simulink model "SecRwLtStBkReclnTrgtPosSelc"  (R2018b)
settings: Solver=FixedStepDiscrete  StartTime=0.0  StopTime=10.0  FixedStep=0.01  RelTol=1e-3
undefined symbols (not defined in the file): KeSMSw4SAcsMd21SecRwLtStBkReclnUpwdDnwdPos_Val, KeSMSw4SAcsMd21SecRwLtStBkReclnUpwdDnwdPosMax_Val, KeSMSw4SAcsMd21SecRwLtStBkReclnUpwdDnwdPosMin_Val, KeSMSw4SAcsMd22SecRwLtStBkReclnUpwdDnwdPos1_Val, KeSMSw4SAcsMd22SecRwLtStBkReclnUpwdDnwdPos1Max_Val, KeSMSw4SAcsMd22SecRwLtStBkReclnUpwdDnwdPos1Min_Val, KeSMSw4SAcsMd22SecRwLtStBkReclnUpwdDnwdPos2_Val, KeSMSw4SAcsMd22SecRwLtStBkReclnUpwdDnwdPos2Max_Val, KeSMSw4SAcsMd22SecRwLtStBkReclnUpwdDnwdPos2Min_Val, KeSMSw4SAcsMd25SecRwLtStBkReclnUpwdDnwdPos_Val, KeSMSw4SAcsMd25SecRwLtStBkReclnUpwdDnwdPosMax_Val, KeSMSw4SAcsMd25SecRwLtStBkReclnUpwdDnwdPosMin_Val, KeSMSw4SAcsMd26SecRwLtStBkReclnUpwdDnwdPos_Val, KeSMSw4SAcsMd26SecRwLtStBkReclnUpwdDnwdPosMax_Val, KeSMSw4SAcsMd26SecRwLtStBkReclnUpwdDnwdPosMin_Val, KeSMSw4sLyingMDSecRwLtStBkReclnUpwdDnwdPos_Val, KeSMSw4sLyingMDSecRwLtStBkReclnUpwdDnwdPosMax_Val, KeSMSw4sLyingMDSecRwLtStBkReclnUpwdDnwdPosMin_Val, KeSMSw4sRecoveryMDSecRwLtStBkReclnUpwdDnwdPos_Val, KeSMSw4sRecoveryMDSecRwLtStBkReclnUpwdDnwdPosMax_Val, KeSMSw4sRecoveryMDSecRwLtStBkReclnUpwdDnwdPosMin_Val, KeSMSw4sVIPMDSecRwLtStBkReclnUpwdDnwdPos_Val, KeSMSw4sVIPMDSecRwLtStBkReclnUpwdDnwdPosMax_Val, KeSMSw4sVIPMDSecRwLtStBkReclnUpwdDnwdPosMin_Val, KeSMSw6sAcsEntrySecRwLtStBkReclnUpwdDnwd1Pos_Val, KeSMSw6sAcsEntrySecRwLtStBkReclnUpwdDnwdPos1Max_Val, KeSMSw6sAcsEntrySecRwLtStBkReclnUpwdDnwdPos1Min_Val, KeSMSw6sAcsEntrySecRwLtStBkReclnUpwdDnwdPos_Val, KeSMSw6sAcsEntrySecRwLtStBkReclnUpwdDnwdPosMax_Val, KeSMSw6sAcsEntrySecRwLtStBkReclnUpwdDnwdPosMin_Val, KeSMSw6sAcsExtSecRwLtStBkReclnUpwdDnwdPos_Val, KeSMSw6sAcsExtSecRwLtStBkReclnUpwdDnwdPosMax_Val, KeSMSw6sAcsExtSecRwLtStBkReclnUpwdDnwdPosMin_Val, KeSMSw6sRecoveryMdSecRwLtStBkReclnUpwdDnwdPos_Val, KeSMSw6sRecoveryMdSecRwLtStBkReclnUpwdDnwdPosMax_Val, KeSMSw6sRecoveryMdSecRwLtStBkReclnUpwdDnwdPosMin_Val, KeSMSw6sVIPSecRwLtStBkReclnUpwdDnwdPos_Val, KeSMSw6sVIPSecRwLtStBkReclnUpwdDnwdPosMax_Val, KeSMSw6sVIPSecRwLtStBkReclnUpwdDnwdPosMin_Val, KeSMSwAcsEntrySecRwLtStBkReclnUpwdDnwdPos1_Val, KeSMSwAcsEntrySecRwLtStBkReclnUpwdDnwdPos1Max_Val, KeSMSwAcsEntrySecRwLtStBkReclnUpwdDnwdPos1Min_Val, KeSMSwAcsEntrySecRwLtStBkReclnUpwdDnwdPos_Val, KeSMSwAcsEntrySecRwLtStBkReclnUpwdDnwdPosMax_Val, KeSMSwAcsEntrySecRwLtStBkReclnUpwdDnwdPosMin_Val, KeSMSwAcsExtSecRwLtStBkReclnUpwdDnwdPos_Val, KeSMSwAcsExtSecRwLtStBkReclnUpwdDnwdPosMax_Val, KeSMSwAcsExtSecRwLtStBkReclnUpwdDnwdPosMin_Val, KeSMSwAcsMd32SecRwLtStBkReclnUpwdDnwdPos1_Val, KeSMSwAcsMd32SecRwLtStBkReclnUpwdDnwdPos1Max_Val, KeSMSwAcsMd32SecRwLtStBkReclnUpwdDnwdPos1Min_Val, KeSMSwAcsMd32SecRwLtStBkReclnUpwdDnwdPos_Val, KeSMSwAcsMd32SecRwLtStBkReclnUpwdDnwdPosMax_Val, KeSMSwAcsMd32SecRwLtStBkReclnUpwdDnwdPosMin_Val, KeSMSwAcsMd8SecRwLtStBkReclnUpwdDnwdPos_Val, KeSMSwAcsMd8SecRwLtStBkReclnUpwdDnwdPosMax_Val, KeSMSwAcsMd8SecRwLtStBkReclnUpwdDnwdPosMin_Val, KeSMSwRecoveryMdSecRwLtStBkReclnUpwdDnwdPos_Val, KeSMSwRecoveryMdSecRwLtStBkReclnUpwdDnwdPosMax_Val, KeSMSwRecoveryMdSecRwLtStBkReclnUpwdDnwdPosMin_Val ... (+3)
libraries: TrgtPosSelcLib x13, StIsPosChkLib x1, simulink x1
(part 2 of 2)

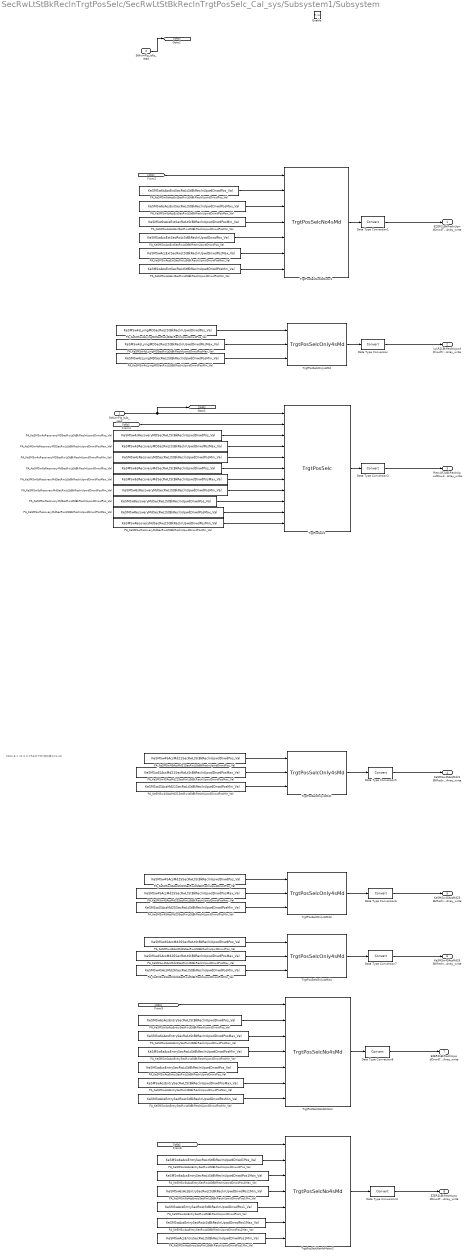
== system SecRwLtStBkReclnTrgtPosSelc/SecRwLtStBkReclnTrgtPosSelc_Cal_sys/Subsystem1/Subsystem ==
  note: 2023.8.1 V2.0.0 CR421790 增加模式21-26
  StNumFlg_Is4s_read : Inport
  StNumFlg_Is6s_read : Inport  Port=2
  Enable : EnablePort
  Data Type Conversion{,1..3,5..8} (8 alike) : DataTypeConversion
  PA_KeSMSw4SAcsMd21SecRwLtStBkReclnUpwdDnwdPosMax_Val : Constant  Value=KeSMSw4SAcsMd21SecRwLtStBkReclnUpwdDnwdPosMax_Val
  PA_KeSMSw4SAcsMd21SecRwLtStBkReclnUpwdDnwdPosMin_Val : Constant  Value=KeSMSw4SAcsMd21SecRwLtStBkReclnUpwdDnwdPosMin_Val
  PA_KeSMSw4SAcsMd21SecRwLtStBkReclnUpwdDnwdPos_Val : Constant  Value=KeSMSw4SAcsMd21SecRwLtStBkReclnUpwdDnwdPos_Val
  PA_KeSMSw4SAcsMd25SecRwLtStBkReclnUpwdDnwdPosMax_Val : Constant  Value=KeSMSw4SAcsMd25SecRwLtStBkReclnUpwdDnwdPosMax_Val
  PA_KeSMSw4SAcsMd25SecRwLtStBkReclnUpwdDnwdPosMin_Val : Constant  Value=KeSMSw4SAcsMd25SecRwLtStBkReclnUpwdDnwdPosMin_Val
  PA_KeSMSw4SAcsMd25SecRwLtStBkReclnUpwdDnwdPos_Val : Constant  Value=KeSMSw4SAcsMd25SecRwLtStBkReclnUpwdDnwdPos_Val
  PA_KeSMSw4SAcsMd26SecRwLtStBkReclnUpwdDnwdPosMax_Val : Constant  Value=KeSMSw4SAcsMd26SecRwLtStBkReclnUpwdDnwdPosMax_Val
  PA_KeSMSw4SAcsMd26SecRwLtStBkReclnUpwdDnwdPosMin_Val : Constant  Value=KeSMSw4SAcsMd26SecRwLtStBkReclnUpwdDnwdPosMin_Val
  PA_KeSMSw4SAcsMd26SecRwLtStBkReclnUpwdDnwdPos_Val : Constant  Value=KeSMSw4SAcsMd26SecRwLtStBkReclnUpwdDnwdPos_Val
  PA_KeSMSw4sLyingMDSecRwLtStBkReclnUpwdDnwdPosMax_Val : Constant  Value=KeSMSw4sLyingMDSecRwLtStBkReclnUpwdDnwdPosMax_Val
  PA_KeSMSw4sLyingMDSecRwLtStBkReclnUpwdDnwdPosMin_Val : Constant  Value=KeSMSw4sLyingMDSecRwLtStBkReclnUpwdDnwdPosMin_Val
  PA_KeSMSw4sLyingMDSecRwLtStBkReclnUpwdDnwdPos_Val : Constant  Value=KeSMSw4sLyingMDSecRwLtStBkReclnUpwdDnwdPos_Val
  PA_KeSMSw4sRecoveryMDSecRwLtStBkReclnUpwdDnwdPosMax_Val : Constant  Value=KeSMSw4sRecoveryMDSecRwLtStBkReclnUpwdDnwdPosMax_Val
  PA_KeSMSw4sRecoveryMDSecRwLtStBkReclnUpwdDnwdPosMin_Val : Constant  Value=KeSMSw4sRecoveryMDSecRwLtStBkReclnUpwdDnwdPosMin_Val
  PA_KeSMSw4sRecoveryMDSecRwLtStBkReclnUpwdDnwdPos_Val : Constant  Value=KeSMSw4sRecoveryMDSecRwLtStBkReclnUpwdDnwdPos_Val
  PA_KeSMSw6sAcsEntrySecRwLtStBkReclnUpwdDnwd1Pos_Val : Constant  Value=KeSMSw6sAcsEntrySecRwLtStBkReclnUpwdDnwd1Pos_Val
  PA_KeSMSw6sAcsEntrySecRwLtStBkReclnUpwdDnwdPos1Max_Val : Constant  Value=KeSMSw6sAcsEntrySecRwLtStBkReclnUpwdDnwdPos1Max_Val
  PA_KeSMSw6sAcsEntrySecRwLtStBkReclnUpwdDnwdPos1Min_Val : Constant  Value=KeSMSw6sAcsEntrySecRwLtStBkReclnUpwdDnwdPos1Min_Val
  PA_KeSMSw6sAcsEntrySecRwLtStBkReclnUpwdDnwdPosMax_Val : Constant  Value=KeSMSw6sAcsEntrySecRwLtStBkReclnUpwdDnwdPosMax_Val
  PA_KeSMSw6sAcsEntrySecRwLtStBkReclnUpwdDnwdPosMin_Val : Constant  Value=KeSMSw6sAcsEntrySecRwLtStBkReclnUpwdDnwdPosMin_Val
  PA_KeSMSw6sAcsEntrySecRwLtStBkReclnUpwdDnwdPos_Val : Constant  Value=KeSMSw6sAcsEntrySecRwLtStBkReclnUpwdDnwdPos_Val
  PA_KeSMSw6sAcsExtSecRwLtStBkReclnUpwdDnwdPosMax_Val : Constant  Value=KeSMSw6sAcsExtSecRwLtStBkReclnUpwdDnwdPosMax_Val
  PA_KeSMSw6sAcsExtSecRwLtStBkReclnUpwdDnwdPosMin_Val : Constant  Value=KeSMSw6sAcsExtSecRwLtStBkReclnUpwdDnwdPosMin_Val
  PA_KeSMSw6sAcsExtSecRwLtStBkReclnUpwdDnwdPos_Val : Constant  Value=KeSMSw6sAcsExtSecRwLtStBkReclnUpwdDnwdPos_Val
  PA_KeSMSw6sRecoveryMdSecRwLtStBkReclnUpwdDnwdPosMax_Val : Constant  Value=KeSMSw6sRecoveryMdSecRwLtStBkReclnUpwdDnwdPosMax_Val
  PA_KeSMSw6sRecoveryMdSecRwLtStBkReclnUpwdDnwdPosMin_Val : Constant  Value=KeSMSw6sRecoveryMdSecRwLtStBkReclnUpwdDnwdPosMin_Val
  PA_KeSMSw6sRecoveryMdSecRwLtStBkReclnUpwdDnwdPos_Val : Constant  Value=KeSMSw6sRecoveryMdSecRwLtStBkReclnUpwdDnwdPos_Val
  PA_KeSMSwAcsEntrySecRwLtStBkReclnUpwdDnwdPos1Max_Val : Constant  Value=KeSMSwAcsEntrySecRwLtStBkReclnUpwdDnwdPos1Max_Val
  PA_KeSMSwAcsEntrySecRwLtStBkReclnUpwdDnwdPos1Min_Val : Constant  Value=KeSMSwAcsEntrySecRwLtStBkReclnUpwdDnwdPos1Min_Val
  PA_KeSMSwAcsEntrySecRwLtStBkReclnUpwdDnwdPos1_Val : Constant  Value=KeSMSwAcsEntrySecRwLtStBkReclnUpwdDnwdPos1_Val
  PA_KeSMSwAcsEntrySecRwLtStBkReclnUpwdDnwdPosMax_Val : Constant  Value=KeSMSwAcsEntrySecRwLtStBkReclnUpwdDnwdPosMax_Val
  PA_KeSMSwAcsEntrySecRwLtStBkReclnUpwdDnwdPosMin_Val : Constant  Value=KeSMSwAcsEntrySecRwLtStBkReclnUpwdDnwdPosMin_Val
  PA_KeSMSwAcsEntrySecRwLtStBkReclnUpwdDnwdPos_Val : Constant  Value=KeSMSwAcsEntrySecRwLtStBkReclnUpwdDnwdPos_Val
  PA_KeSMSwAcsExtSecRwLtStBkReclnUpwdDnwdPosMax_Val : Constant  Value=KeSMSwAcsExtSecRwLtStBkReclnUpwdDnwdPosMax_Val
  PA_KeSMSwAcsExtSecRwLtStBkReclnUpwdDnwdPosMin_Val : Constant  Value=KeSMSwAcsExtSecRwLtStBkReclnUpwdDnwdPosMin_Val
  PA_KeSMSwAcsExtSecRwLtStBkReclnUpwdDnwdPos_Val : Constant  Value=KeSMSwAcsExtSecRwLtStBkReclnUpwdDnwdPos_Val
  PA_KeSMSwRecoveryMdSecRwLtStBkReclnUpwdDnwdPosMax_Val : Constant  Value=KeSMSwRecoveryMdSecRwLtStBkReclnUpwdDnwdPosMax_Val
  PA_KeSMSwRecoveryMdSecRwLtStBkReclnUpwdDnwdPosMin_Val : Constant  Value=KeSMSwRecoveryMdSecRwLtStBkReclnUpwdDnwdPosMin_Val
  PA_KeSMSwRecoveryMdSecRwLtStBkReclnUpwdDnwdPos_Val : Constant  Value=KeSMSwRecoveryMdSecRwLtStBkReclnUpwdDnwdPos_Val
  TrgtPosSelc1 : TrgtPosSelcLib/TrgtPosSelc  SystemSampleTime=-1
  TrgtPosSelcNot4sMotor : TrgtPosSelcLib/TrgtPosSelcNo4sMd  SystemSampleTime=-1
  TrgtPosSelcNot4sMotor1 : TrgtPosSelcLib/TrgtPosSelcNo4sMd  SystemSampleTime=-1
  TrgtPosSelcNot4sMotor2 : TrgtPosSelcLib/TrgtPosSelcNo4sMd  SystemSampleTime=-1
  TrgtPosSelcOnly4sMd{,1,3..4} (4 alike) : TrgtPosSelcLib/TrgtPosSelcOnly4sMd  SystemSampleTime=-1
  EZQR2LBkReclnUpwdDnwdTrgtPosCalib_TrgtPosArray_write : Outport
      settings: EnsureOutportIsVirtual=on
  LyLR2LBkReclnUpwdDnwdTrgtPosCalib_TrgtPosArray_write : Outport  Port=2
  RecvLR2LBkReclnUpwdDnwdTrgtPosCalib_TrgtPosArray_write : Outport  Port=3
      settings: EnsureOutportIsVirtual=on
  KeSMSw4SAcsMd21BkReclnUpwdDnwdTrgtPosCalib_TrgtPosArray_write : Outport  Port=4  InitialOutput=0
  KeSMSw4SAcsMd25BkReclnUpwdDnwdTrgtPosCalib_TrgtPosArray_write : Outport  Port=5  InitialOutput=0
  KeSMSw4SAcsMd26BkReclnUpwdDnwdTrgtPosCalib_TrgtPosArray_write : Outport  Port=6  InitialOutput=0
  EZER2LBkReclnUpwdDnwdTrgtPosCalib_TrgtPosArray_write : Outport  Port=7
  EZER2LBkReclnUpwdDnwdTrgtPosCalib1_TrgtPosArray_write : Outport  Port=8
  wires:
  [is6s] -> TrgtPosSelcNot4sMotor1/1
  PA_KeSMSw4sLyingMDSecRwLtStBkReclnUpwdDnwdPosMax_Val/1 -> TrgtPosSelcOnly4sMd/2
  PA_KeSMSwAcsExtSecRwLtStBkReclnUpwdDnwdPosMin_Val/1 -> TrgtPosSelcNot4sMotor1/7
  PA_KeSMSw4sLyingMDSecRwLtStBkReclnUpwdDnwdPos_Val/1 -> TrgtPosSelcOnly4sMd/1
  TrgtPosSelcOnly4sMd/1 -> Data Type Conversion/1
  StNumFlg_Is4s_read/1 -> [is4s], TrgtPosSelc1/1
  PA_KeSMSw6sAcsExtSecRwLtStBkReclnUpwdDnwdPos_Val/1 -> TrgtPosSelcNot4sMotor1/2
  PA_KeSMSw4sRecoveryMDSecRwLtStBkReclnUpwdDnwdPosMax_Val/1 -> TrgtPosSelc1/4
  PA_KeSMSw4sLyingMDSecRwLtStBkReclnUpwdDnwdPosMin_Val/1 -> TrgtPosSelcOnly4sMd/3
  PA_KeSMSw4sRecoveryMDSecRwLtStBkReclnUpwdDnwdPos_Val/1 -> TrgtPosSelc1/3
  PA_KeSMSw6sAcsExtSecRwLtStBkReclnUpwdDnwdPosMin_Val/1 -> TrgtPosSelcNot4sMotor1/4
  StNumFlg_Is6s_read/1 -> [is6s]
  PA_KeSMSwAcsExtSecRwLtStBkReclnUpwdDnwdPosMax_Val/1 -> TrgtPosSelcNot4sMotor1/6
  PA_KeSMSw6sAcsExtSecRwLtStBkReclnUpwdDnwdPosMax_Val/1 -> TrgtPosSelcNot4sMotor1/3
  PA_KeSMSw6sRecoveryMdSecRwLtStBkReclnUpwdDnwdPos_Val/1 -> TrgtPosSelc1/6
  PA_KeSMSw6sRecoveryMdSecRwLtStBkReclnUpwdDnwdPosMin_Val/1 -> TrgtPosSelc1/8
  PA_KeSMSwRecoveryMdSecRwLtStBkReclnUpwdDnwdPosMax_Val/1 -> TrgtPosSelc1/10
  TrgtPosSelc1/1 -> Data Type Conversion3/1
  TrgtPosSelcNot4sMotor1/1 -> Data Type Conversion1/1
  [is6s] -> TrgtPosSelc1/2
  PA_KeSMSwAcsExtSecRwLtStBkReclnUpwdDnwdPos_Val/1 -> TrgtPosSelcNot4sMotor1/5
  PA_KeSMSwRecoveryMdSecRwLtStBkReclnUpwdDnwdPosMin_Val/1 -> TrgtPosSelc1/11
  PA_KeSMSw6sRecoveryMdSecRwLtStBkReclnUpwdDnwdPosMax_Val/1 -> TrgtPosSelc1/7
  PA_KeSMSw4sRecoveryMDSecRwLtStBkReclnUpwdDnwdPosMin_Val/1 -> TrgtPosSelc1/5
  PA_KeSMSwRecoveryMdSecRwLtStBkReclnUpwdDnwdPos_Val/1 -> TrgtPosSelc1/9
  Data Type Conversion/1 -> LyLR2LBkReclnUpwdDnwdTrgtPosCalib_TrgtPosArray_write/1
  TrgtPosSelcOnly4sMd1/1 -> Data Type Conversion5/1
  TrgtPosSelcOnly4sMd3/1 -> Data Type Conversion6/1
  TrgtPosSelcOnly4sMd4/1 -> Data Type Conversion7/1
  PA_KeSMSw4SAcsMd21SecRwLtStBkReclnUpwdDnwdPosMin_Val/1 -> TrgtPosSelcOnly4sMd1/3
  PA_KeSMSw4SAcsMd21SecRwLtStBkReclnUpwdDnwdPosMax_Val/1 -> TrgtPosSelcOnly4sMd1/2
  PA_KeSMSw4SAcsMd21SecRwLtStBkReclnUpwdDnwdPos_Val/1 -> TrgtPosSelcOnly4sMd1/1
  PA_KeSMSw4SAcsMd26SecRwLtStBkReclnUpwdDnwdPos_Val/1 -> TrgtPosSelcOnly4sMd4/1
  PA_KeSMSw4SAcsMd26SecRwLtStBkReclnUpwdDnwdPosMax_Val/1 -> TrgtPosSelcOnly4sMd4/2
  PA_KeSMSw4SAcsMd26SecRwLtStBkReclnUpwdDnwdPosMin_Val/1 -> TrgtPosSelcOnly4sMd4/3
  PA_KeSMSw4SAcsMd25SecRwLtStBkReclnUpwdDnwdPos_Val/1 -> TrgtPosSelcOnly4sMd3/1
  PA_KeSMSw4SAcsMd25SecRwLtStBkReclnUpwdDnwdPosMax_Val/1 -> TrgtPosSelcOnly4sMd3/2
  PA_KeSMSw4SAcsMd25SecRwLtStBkReclnUpwdDnwdPosMin_Val/1 -> TrgtPosSelcOnly4sMd3/3
  Data Type Conversion1/1 -> EZQR2LBkReclnUpwdDnwdTrgtPosCalib_TrgtPosArray_write/1
  Data Type Conversion3/1 -> RecvLR2LBkReclnUpwdDnwdTrgtPosCalib_TrgtPosArray_write/1
  Data Type Conversion5/1 -> KeSMSw4SAcsMd21BkReclnUpwdDnwdTrgtPosCalib_TrgtPosArray_write/1
  Data Type Conversion6/1 -> KeSMSw4SAcsMd25BkReclnUpwdDnwdTrgtPosCalib_TrgtPosArray_write/1
  Data Type Conversion7/1 -> KeSMSw4SAcsMd26BkReclnUpwdDnwdTrgtPosCalib_TrgtPosArray_write/1
  Data Type Conversion8/1 -> EZER2LBkReclnUpwdDnwdTrgtPosCalib_TrgtPosArray_write/1
  [is6s] -> TrgtPosSelcNot4sMotor2/1
  PA_KeSMSw6sAcsEntrySecRwLtStBkReclnUpwdDnwdPos1Min_Val/1 -> TrgtPosSelcNot4sMotor2/4
  PA_KeSMSwAcsEntrySecRwLtStBkReclnUpwdDnwdPos1Min_Val/1 -> TrgtPosSelcNot4sMotor2/7
  PA_KeSMSwAcsEntrySecRwLtStBkReclnUpwdDnwdPos1_Val/1 -> TrgtPosSelcNot4sMotor2/5
  PA_KeSMSw6sAcsEntrySecRwLtStBkReclnUpwdDnwd1Pos_Val/1 -> TrgtPosSelcNot4sMotor2/2
  PA_KeSMSwAcsEntrySecRwLtStBkReclnUpwdDnwdPos1Max_Val/1 -> TrgtPosSelcNot4sMotor2/6
  [is6s] -> TrgtPosSelcNot4sMotor/1
  TrgtPosSelcNot4sMotor/1 -> Data Type Conversion8/1
  PA_KeSMSw6sAcsEntrySecRwLtStBkReclnUpwdDnwdPos1Max_Val/1 -> TrgtPosSelcNot4sMotor2/3
  PA_KeSMSwAcsEntrySecRwLtStBkReclnUpwdDnwdPosMax_Val/1 -> TrgtPosSelcNot4sMotor/6
  PA_KeSMSw6sAcsEntrySecRwLtStBkReclnUpwdDnwdPosMin_Val/1 -> TrgtPosSelcNot4sMotor/4
  PA_KeSMSwAcsEntrySecRwLtStBkReclnUpwdDnwdPos_Val/1 -> TrgtPosSelcNot4sMotor/5
  PA_KeSMSwAcsEntrySecRwLtStBkReclnUpwdDnwdPosMin_Val/1 -> TrgtPosSelcNot4sMotor/7
  PA_KeSMSw6sAcsEntrySecRwLtStBkReclnUpwdDnwdPosMax_Val/1 -> TrgtPosSelcNot4sMotor/3
  TrgtPosSelcNot4sMotor2/1 -> Data Type Conversion2/1
  PA_KeSMSw6sAcsEntrySecRwLtStBkReclnUpwdDnwdPos_Val/1 -> TrgtPosSelcNot4sMotor/2
  Data Type Conversion2/1 -> EZER2LBkReclnUpwdDnwdTrgtPosCalib1_TrgtPosArray_write/1

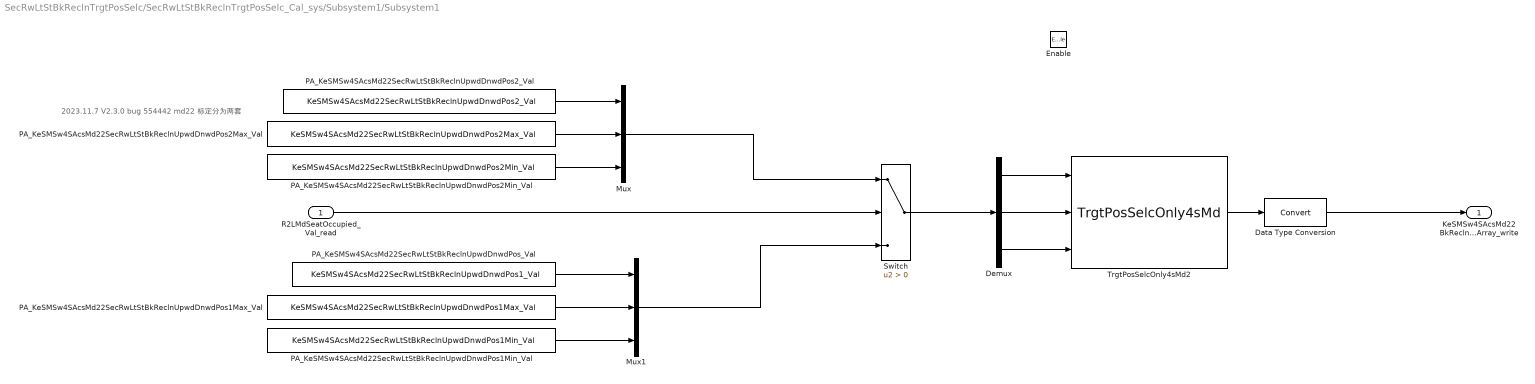
== system SecRwLtStBkReclnTrgtPosSelc/SecRwLtStBkReclnTrgtPosSelc_Cal_sys/Subsystem1/Subsystem1 ==
  note: 2023.11.7 V2.3.0 bug 554442 md22 标定分为两套
  R2LMdSeatOccupied_Val_read : Inport
  Enable : EnablePort
  Data Type Conversion : DataTypeConversion
  Demux : Demux  Outputs=3
  Mux : Mux  Inputs=3
  Mux1 : Mux  Inputs=3
  PA_KeSMSw4SAcsMd22SecRwLtStBkReclnUpwdDnwdPos1Max_Val : Constant  Value=KeSMSw4SAcsMd22SecRwLtStBkReclnUpwdDnwdPos1Max_Val
  PA_KeSMSw4SAcsMd22SecRwLtStBkReclnUpwdDnwdPos1Min_Val : Constant  Value=KeSMSw4SAcsMd22SecRwLtStBkReclnUpwdDnwdPos1Min_Val
  PA_KeSMSw4SAcsMd22SecRwLtStBkReclnUpwdDnwdPos2Max_Val : Constant  Value=KeSMSw4SAcsMd22SecRwLtStBkReclnUpwdDnwdPos2Max_Val
  PA_KeSMSw4SAcsMd22SecRwLtStBkReclnUpwdDnwdPos2Min_Val : Constant  Value=KeSMSw4SAcsMd22SecRwLtStBkReclnUpwdDnwdPos2Min_Val
  PA_KeSMSw4SAcsMd22SecRwLtStBkReclnUpwdDnwdPos2_Val : Constant  Value=KeSMSw4SAcsMd22SecRwLtStBkReclnUpwdDnwdPos2_Val
  PA_KeSMSw4SAcsMd22SecRwLtStBkReclnUpwdDnwdPos_Val : Constant  Value=KeSMSw4SAcsMd22SecRwLtStBkReclnUpwdDnwdPos1_Val
  Switch : Switch  Criteria=u2 > Threshold
  TrgtPosSelcOnly4sMd2 : TrgtPosSelcLib/TrgtPosSelcOnly4sMd  SystemSampleTime=-1
  KeSMSw4SAcsMd22BkReclnUpwdDnwdTrgtPosCalib_TrgtPosArray_write : Outport  InitialOutput=0
  wires:
  TrgtPosSelcOnly4sMd2/1 -> Data Type Conversion/1
  R2LMdSeatOccupied_Val_read/1 -> Switch/2
  Data Type Conversion/1 -> KeSMSw4SAcsMd22BkReclnUpwdDnwdTrgtPosCalib_TrgtPosArray_write/1
  PA_KeSMSw4SAcsMd22SecRwLtStBkReclnUpwdDnwdPos2Min_Val/1 -> Mux/3
  PA_KeSMSw4SAcsMd22SecRwLtStBkReclnUpwdDnwdPos2Max_Val/1 -> Mux/2
  PA_KeSMSw4SAcsMd22SecRwLtStBkReclnUpwdDnwdPos2_Val/1 -> Mux/1
  Mux/1 -> Switch/1
  PA_KeSMSw4SAcsMd22SecRwLtStBkReclnUpwdDnwdPos1Min_Val/1 -> Mux1/3
  PA_KeSMSw4SAcsMd22SecRwLtStBkReclnUpwdDnwdPos1Max_Val/1 -> Mux1/2
  PA_KeSMSw4SAcsMd22SecRwLtStBkReclnUpwdDnwdPos_Val/1 -> Mux1/1
  Mux1/1 -> Switch/3
  Switch/1 -> Demux/1
  Demux/2 -> TrgtPosSelcOnly4sMd2/2
  Demux/1 -> TrgtPosSelcOnly4sMd2/1
  Demux/3 -> TrgtPosSelcOnly4sMd2/3

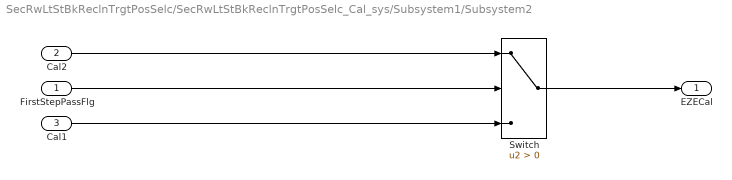
== system SecRwLtStBkReclnTrgtPosSelc/SecRwLtStBkReclnTrgtPosSelc_Cal_sys/Subsystem1/Subsystem2 ==
  FirstStepPassFlg : Inport
  Cal2 : Inport  Port=2
  Cal1 : Inport  Port=3
  Switch : Switch  Criteria=u2 > Threshold
  EZECal : Outport
  wires:
  Switch/1 -> EZECal/1
  FirstStepPassFlg/1 -> Switch/2
  Cal2/1 -> Switch/1
  Cal1/1 -> Switch/3
